simulink model "FilterChain"  (R2025b)
settings: Solver=VariableStepAuto  StartTime=0.0  StopTime=10.0  RelTol=1e-3
values from neighbouring files (symbols this model uses):
  compFilt = design(compSpec,'SystemObject',true)    [FilterChainDesign.m]
  finalFilt = design(finalSpec,'equiripple','SystemObject',true)    [FilterChainDesign.m]
  hbFilt = design(hbSpec,'SystemObject',true)    [FilterChainDesign.m]
libraries: dsphdlfiltering2 x4, dsphdlsigops2 x1
settings Model: Creator=aidan  LastModifiedBy=aidan
settings DebuggingCC: SingleTaskRateTransMsg=error

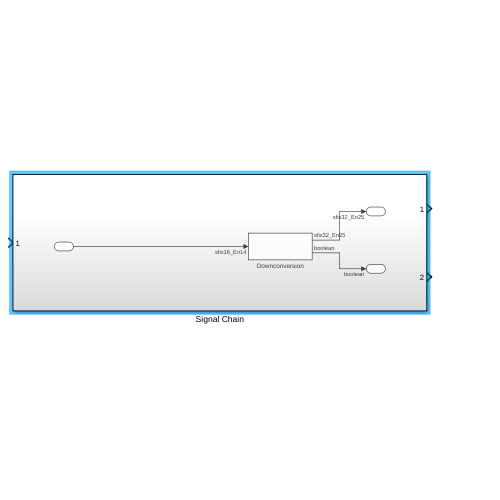
[thumbnail: Simulink's stored preview of the top-level diagram]
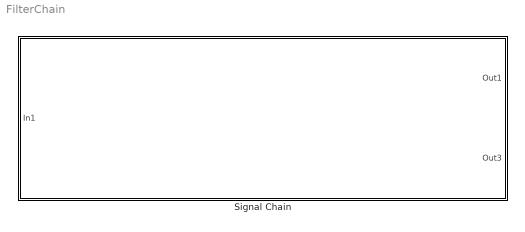
== system FilterChain ==
  Signal Chain : Subsystem

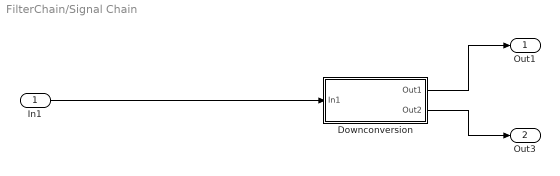
== system FilterChain/Signal Chain ==
  In1 : Inport
  Downconversion : Subsystem
  Out1 : Outport
  Out3 : Outport  Port=2
  wires:
  Downconversion/1(Out1) -> Out1/1
  Downconversion/2(Out2) -> Out3/1
  In1/1 -> Downconversion/1(In1)

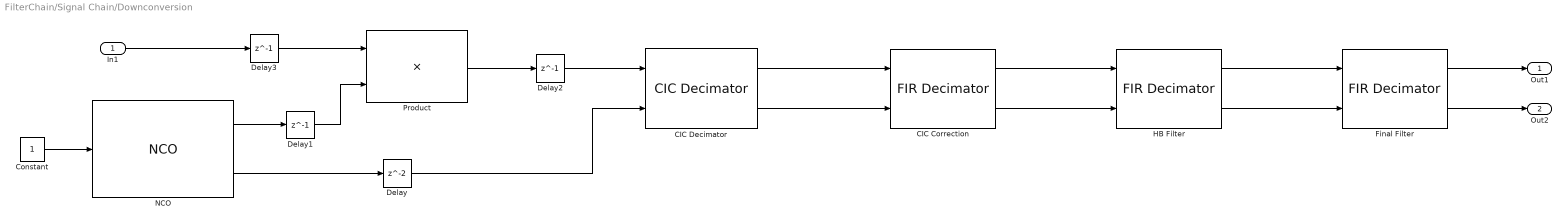
== system FilterChain/Signal Chain/Downconversion ==
  In1 : Inport
  CIC Correction : dsphdlfiltering2/FIR Decimator  NumeratorSource=Property  Numerator=compFilt.Numerator  NumeratorPrototype=[]  FilterStructure=Direct form systolic  DecimationFactor=compFilt.DecimationFactor  NumCycles=500  OptimizeSymmCoeff=on  SimulateUsing=Code generation  roundingMode=Floor  overflowMode=off  CoefficientsDataTypeStr=Inherit: Same word length as input  OutputDataTypeStr=Inherit: Same word length as input  ResetInputPort=off  HDLGlobalReset=on
  CIC Decimator : dsphdlfiltering2/CIC Decimator  DecimationSource=Property  DecimationFactor=cicParams.DecimationFactor  MaxDecimationFactor=2  DifferentialDelay=cicParams.DifferentialDelay  NumSections=cicParams.NumSections  GainCorrection=on  SimulateUsing=Code generation  OutputDataType=Same word length as input  OutputWordLength=16  ResetInputPort=off  HDLGlobalReset=on
  Constant : Constant  OutDataTypeStr=boolean
  Delay : Delay  InitialCondition=0
  Delay1 : Delay  DelayLength=1  InitialCondition=0
  Delay2 : Delay  DelayLength=1  InitialCondition=0
  Delay3 : Delay  DelayLength=1  InitialCondition=0
  Final Filter : dsphdlfiltering2/FIR Decimator  NumeratorSource=Property  Numerator=finalFilt.Numerator  NumeratorPrototype=[]  FilterStructure=Direct form systolic  DecimationFactor=finalFilt.DecimationFactor  NumCycles=2000  OptimizeSymmCoeff=on  SimulateUsing=Code generation  roundingMode=Floor  overflowMode=off  CoefficientsDataTypeStr=Inherit: Same word length as input  OutputDataTypeStr=Inherit: Same word length as input  ResetInputPort=off  HDLGlobalReset=on
  HB Filter : dsphdlfiltering2/FIR Decimator  NumeratorSource=Property  Numerator=hbFilt.Numerator  NumeratorPrototype=[]  FilterStructure=Direct form systolic  DecimationFactor=hbFilt.DecimationFactor  NumCycles=1000  OptimizeSymmCoeff=on  SimulateUsing=Code generation  roundingMode=Floor  overflowMode=off  CoefficientsDataTypeStr=Inherit: Same word length as input  OutputDataTypeStr=Inherit: Same word length as input  ResetInputPort=off  HDLGlobalReset=on
  NCO : dsphdlsigops2/NCO  PhaseIncrementSource=Property  PhaseIncrement=nco.PhaseInc  PhaseOffsetSource=Property  PhaseOffset=0  DitherSource=Property  NumDitherBits=nco.NumDitherBits  SamplesPerFrame=1  LUTCompress=off  ResetAction=off  Waveform=Complex exponential  PhasePort=off  SimulateUsing=Code generation  AccumulatorWL=nco.AccWL  PhaseQuantization=on  NumQuantizerAccumulatorBits=nco.QuantAccWL  OutputDataType=Binary point scaling  OutputWL=16  OutputFL=14
      settings: LibrarySourceBlock=dsphdlsrcs2/NCO
  Product : Product  InputSameDT=on
  Out1 : Outport
  Out2 : Outport  Port=2
  wires:
  NCO/2 -> Delay/1
  Delay/1 -> CIC Decimator/2
  NCO/1 -> Delay1/1
  Delay1/1 -> Product/2
  Product/1 -> Delay2/1
  Delay2/1 -> CIC Decimator/1
  CIC Decimator/2 -> CIC Correction/2
  CIC Decimator/1 -> CIC Correction/1
  CIC Correction/2 -> HB Filter/2
  CIC Correction/1 -> HB Filter/1
  HB Filter/2 -> Final Filter/2
  HB Filter/1 -> Final Filter/1
  In1/1 -> Delay3/1
  Delay3/1 -> Product/1
  Constant/1 -> NCO/1
  Final Filter/1 -> Out1/1
  Final Filter/2 -> Out2/1
